simulink subsystem "ScanDc"  (R2025a)
settings: Solver=VariableStepAuto  StartTime=0.0  StopTime=10.0  RelTol=1e-3
model mask{F0=0, Theta0=0, Kp_LF=0, Ki_LF=0, Ts=0, Amplitudedc=scan.Vdc, Amplitude=0, Amplitude1=0, voltagedc=HVDC.Vdc, voltage=0, mva=0, f=scan.f, Tdis=scan.start, Tend=scan.end, T=1/scan.samplingfrequency}
  mask prompts: F0 "Initial frequency (Hz)"; Theta0 "Inital angle (deg)"; Kp_LF "Proportional gain"; Ki_LF "Integral gain"; Ts "Sample time (sec)"; Amplitudedc "DC voltage disturbance (PU)"; Amplitude "D axis voltage disturbance (PU)"; Amplitude1 "Q axis voltage disturbance (PU)"; voltagedc "Base DC Voltage (V)"; voltage "Base AC Voltage (V)"; mva "Base voltr ampere (VA)"; f "Disturbance Frequency (Hz)"; Tdis "Disturbance start time (sec)"; Tend "Disturbance end time (sec)"; T "Sample Time of PRBS (sec)"
undefined symbols (not defined in the file): DiscIntNeverNeededParam, ee_sli_rtmsupport, gcbh, w
libraries: slctrl_fre x6, eeGeneralControl x4, slctrl_signal x3, eeTransforms x2, ee_lib x1, nesl_utility x1, simulink x1
(part 1 of 2)
settings Model: Creator=rajarshd  LastModifiedBy=rajarshd

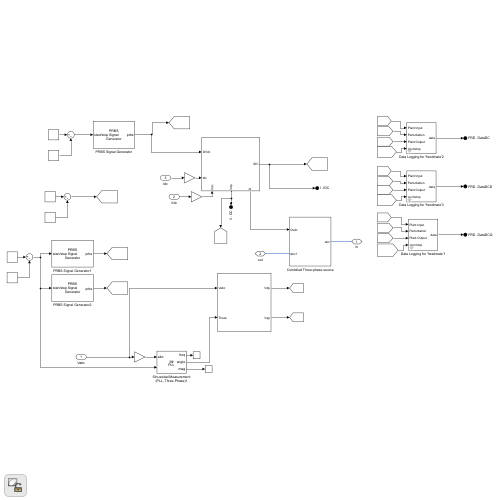
[thumbnail: Simulink's stored preview of the top-level diagram]
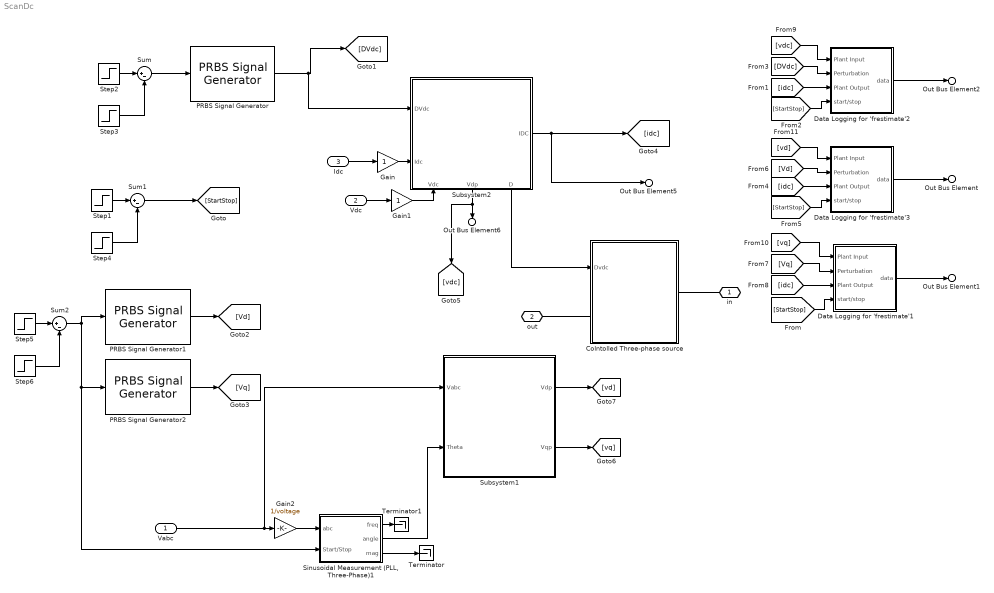
== system ScanDc ==
  Vabc : Inport
  Vdc : Inport  Port=2
  Idc : Inport  Port=3
  Colntolled Three-phase source : Subsystem
  Data Logging for 'frestimate'1 : Subsystem  mask(Companion Data Logger){Ts=T, SignalType=PRBS, Frequencies=[1:1:2e3], NumOfSetPeriod=1, NumOfEstPeriod=1, PRBSNumOfPeriod=1, ReadySignalActiveChoice=VariantPRBS, InfoSignalActiveChoice=VariantPRBS}
      mask prompts: Ts "Sample Time (Ts)"; SignalType "Input Signal Type"; Frequencies "Frequencies Vector"; NumOfSetPeriod "Number of Settling Periods"; NumOfEstPeriod "Number of Estimation Periods"; PRBSNumOfPeriod "Number of PRBS Signal Periods"; ReadySignalActiveChoice "Simulink:Variants:LabelComboBox"; InfoSignalActiveChoice "Simulink:Variants:LabelComboBox"
      mask help: Log data from signal generator blocks to work with "frestimate" API or frequency response estimation.
      mask init:
      | IsSinestreamSignal = strcmpi(get_param(gcb,'SignalType'),'Sinestream');
      |     IsPRBSSignal = strcmpi(get_param(gcb,'SignalType'),'PRBS');
      |     maskObj = Simulink.Mask.get(gcb);
      |     objectSinestream = maskObj.getDialogControl('SinestreamPanel');
      |     objectPRBS = maskObj.getDialogControl('PRBSPanel');
      |     %% Update optional inports
      |     inport_name = {'Frequency Index'};
      |     AvailableBlocks = get_param(gcb,'Blocks');
      |     % what exists in the block (old)
      |     type_in_block = ismember(inport_name,AvailableBlocks);
      |     % what is specified in the dialog (new)
      |     type_in_mask = IsSinestreamSignal;
      |     if IsSinestreamSignal
      |         objectSinestream.Visible = 'on';
      |         objectPRBS.Visible = 'off';
      |         set_param(gcb,'ReadySignalActiveChoice','VariantSinestream');  
      |         set_param(gcb,'InfoSignalActiveChoice','VariantSinestream');        
      |     elseif IsPRBSSignal
      |         objectSinestream.Visible = 'off';
      |         objectPRBS.Visible = 'on';
      |         set_param(gcb,'ReadySignalActiveChoice','VariantPRBS');  
      |         set_param(gcb,'InfoSignalActiveChoice','VariantPRBS');        
      |     end
      |     % Update Inport
      |     port = 5;
      |     port = slctrlblkdlgs.OnlinePIDTuner.utilUpdateInport(gcb,'RateTransition_idx',AvailableBlocks,type_in_mask,type_in_block,1,'Frequency Index',port,1,'Frequencies','double');
      mask TypeOptions SignalType: Sinestream | PRBS
      mask TypeOptions ReadySignalActiveChoice: Generate Ready Signal/LabelModeActiveChoice
      mask TypeOptions InfoSignalActiveChoice: Generate Info Signal/LabelModeActiveChoice
      mask DialogControl Container3 Prompt: Signal Specific Settings
      mask DialogControl ReadySignalActiveChoice Prompt: Label mode active choice:
      mask DialogControl InfoSignalActiveChoice Prompt: Label mode active choice:
  Data Logging for 'frestimate'2 : Subsystem  mask(Companion Data Logger){Ts=T, SignalType=PRBS, Frequencies=[1:1:2e3], NumOfSetPeriod=1, NumOfEstPeriod=1, PRBSNumOfPeriod=1, ReadySignalActiveChoice=VariantPRBS, InfoSignalActiveChoice=VariantPRBS}
      mask prompts: Ts "Sample Time (Ts)"; SignalType "Input Signal Type"; Frequencies "Frequencies Vector"; NumOfSetPeriod "Number of Settling Periods"; NumOfEstPeriod "Number of Estimation Periods"; PRBSNumOfPeriod "Number of PRBS Signal Periods"; ReadySignalActiveChoice "Simulink:Variants:LabelComboBox"; InfoSignalActiveChoice "Simulink:Variants:LabelComboBox"
      mask help: Log data from signal generator blocks to work with "frestimate" API or frequency response estimation.
      mask init: same as ScanDc/Data Logging for 'frestimate'1
      mask TypeOptions SignalType: Sinestream | PRBS
      mask TypeOptions ReadySignalActiveChoice: Generate Ready Signal/LabelModeActiveChoice
      mask TypeOptions InfoSignalActiveChoice: Generate Info Signal/LabelModeActiveChoice
      mask DialogControl Container3 Prompt: Signal Specific Settings
      mask DialogControl ReadySignalActiveChoice Prompt: Label mode active choice:
      mask DialogControl InfoSignalActiveChoice Prompt: Label mode active choice:
  Data Logging for 'frestimate'3 : Subsystem  mask(Companion Data Logger){Ts=T, SignalType=PRBS, Frequencies=[1:1:2e3], NumOfSetPeriod=1, NumOfEstPeriod=1, PRBSNumOfPeriod=1, ReadySignalActiveChoice=VariantPRBS, InfoSignalActiveChoice=VariantPRBS}
      mask prompts: Ts "Sample Time (Ts)"; SignalType "Input Signal Type"; Frequencies "Frequencies Vector"; NumOfSetPeriod "Number of Settling Periods"; NumOfEstPeriod "Number of Estimation Periods"; PRBSNumOfPeriod "Number of PRBS Signal Periods"; ReadySignalActiveChoice "Simulink:Variants:LabelComboBox"; InfoSignalActiveChoice "Simulink:Variants:LabelComboBox"
      mask help: Log data from signal generator blocks to work with "frestimate" API or frequency response estimation.
      mask init: same as ScanDc/Data Logging for 'frestimate'1
      mask TypeOptions SignalType: Sinestream | PRBS
      mask TypeOptions ReadySignalActiveChoice: Generate Ready Signal/LabelModeActiveChoice
      mask TypeOptions InfoSignalActiveChoice: Generate Info Signal/LabelModeActiveChoice
      mask DialogControl Container3 Prompt: Signal Specific Settings
      mask DialogControl ReadySignalActiveChoice Prompt: Label mode active choice:
      mask DialogControl InfoSignalActiveChoice Prompt: Label mode active choice:
  Gain : Gain
  Gain1 : Gain
  Gain2 : Gain  Gain=1/voltage
  PRBS Signal Generator : slctrl_signal/PRBS Signal Generator  DiscreteTs=T  BlockDataType=double  SignalSource=Block parameters  Frequencies=f*2*pi  FreqUnits=rad/s  Amplitudes=Amplitudedc*voltagedc+1e-9  NumOfFreq=3  NumOfPRBSPeriod=1  UseAutogenNumOfPRBSPeriod=off  PRBSSignalOrder=16  UseAutogenPRBSSignalOrder=on  UseExternalTs=off  CompiledTsChoice=InternalTs
      settings: LibrarySourceBlock=slctrlblks/Signal Generation/PRBS Signal Generator
  PRBS Signal Generator1 : slctrl_signal/PRBS Signal Generator  DiscreteTs=T  BlockDataType=double  SignalSource=Block parameters  Frequencies=f*2*pi  FreqUnits=rad/s  Amplitudes=Amplitude*voltage+1e-9  NumOfFreq=3  NumOfPRBSPeriod=1  UseAutogenNumOfPRBSPeriod=off  PRBSSignalOrder=16  UseAutogenPRBSSignalOrder=on  UseExternalTs=off  CompiledTsChoice=InternalTs
      settings: LibrarySourceBlock=slctrlblks/Signal Generation/PRBS Signal Generator
  PRBS Signal Generator2 : slctrl_signal/PRBS Signal Generator  DiscreteTs=T  BlockDataType=double  SignalSource=Block parameters  Frequencies=f*2*pi  FreqUnits=rad/s  Amplitudes=Amplitude1*voltage+1e-9  NumOfFreq=3  NumOfPRBSPeriod=1  UseAutogenNumOfPRBSPeriod=off  PRBSSignalOrder=16  UseAutogenPRBSSignalOrder=on  UseExternalTs=off  CompiledTsChoice=InternalTs
      settings: LibrarySourceBlock=slctrlblks/Signal Generation/PRBS Signal Generator
  "Sinusoidal Measurement (PLL, Three-Phase)1" : Subsystem  LoadFcn=ee_sli_rtmsupport( 'loadfcn', gcbh );  mask(Sinusoidal Measurement (PLL, Three-Phase)){Kp_LF=Kp_LF, Ki_LF=Ki_LF, F0=F0, Theta0=Theta0, Ts=Ts}
      mask prompts: Kp_LF "physmod:ee:library:comments:control:eeSinusoidalMeasurement:LoopFilterProportionalGain_MP"; Ki_LF "physmod:ee:library:comments:control:eeSinusoidalMeasurement:LoopFilterIntegralGain_MP"; F0 "physmod:ee:library:comments:control:eeSinusoidalMeasurement:InitialFrequencyHz_MP"; Theta0 "physmod:ee:library:comments:control:eeSinusoidalMeasurement:InitialPhaseAnglerad_MP"; Ts "physmod:ee:library:comments:control:eeSinusoidalMeasurement:SampleTime1ForInherited_MP"
      mask help: physmod:ee:library:comments:control:eeSinusoidalMeasurement:SinusoidalPowerMeasurementPLLThreePhase_MD
      mask init:
      | timeDomain = ee.mask.initializeThreePhaseSinusoidalMeasurementPLL(Ts);
      settings: CopyFcn=ee_sli_rtmsupport( 'copyfcn', gcbh );  DeleteFcn=ee_sli_rtmsupport( 'deletefcn', gcbh );  ModelCloseFcn=ee_sli_rtmsupport( 'modelclosefcn', gcbh );  PostSaveFcn=ee_sli_rtmsupport( 'postsavefcn', gcbh );  PreCopyFcn=ee_sli_rtmsupport( 'precopyfcn', gcbh );  OpenFcn=ee_sli_rtmsupport( 'openfcn', gcbh );  CloseFcn=ee_sli_rtmsupport( 'closefcn', gcbh );  PreDeleteFcn=ee_sli_rtmsupport( 'predeletefcn', gcbh );
      settings: LibrarySourceBlock=|
      | ee_sl_lib/Measurements/Sinusoidal Measurement
      | (PLL, Three-Phase)
      mask Help: web(nesl_help(gcbh))
      mask TypeOptions Ts:
      | Angle/Integrator with
      | Wrapped State
      | (Discrete or Continuous)/Ts | PI/Integrator
      | (Discrete or Continuous)/Ts | Moving Average
      | (Variable Frequency)/Ts | Low-Pass Filter
      | (Discrete or Continuous)/Ts
      mask DialogControl Kp_LF Prompt: Loop filter proportional gain
      mask DialogControl Ki_LF Prompt: Loop filter integral gain
      mask DialogControl F0 Prompt: Initial frequency (Hz)
      mask DialogControl Theta0 Prompt: Initial phase angle (rad)
      mask DialogControl Ts Prompt: Sample time (-1 for inherited)
      mask Display: ee.mask.drawThreePhaseSinusoidalMeasurementPLL;
  Step1 : Step  Time=Tdis-0.001  SampleTime=Ts
  Step2 : Step  Time=Tdis  SampleTime=Ts
  Step3 : Step  Time=Tend  SampleTime=Ts
  Step4 : Step  Time=Tend-0.001  SampleTime=Ts
  Step5 : Step  Time=Tdis  SampleTime=Ts
  Step6 : Step  Time=Tend  SampleTime=Ts
  Subsystem1 : Subsystem
      settings: PortSchema="{\"entries\":[{\"content\":{\"sides\":[{\"content\":{},\"type\":\"ConnectorPlacement.EquallySpacedRectSide\",\"uuid\":\"9594ab20-6a90-4061-9191-964719779161\"},{\"content\":{\"side\":\"RIGHT\"},\"type\":\"ConnectorPlacement.EquallySpacedRectSide\",\"uuid\":\"7728c146-30c2-48f5-81ca-653b56ee64fb\"},{\"content\":{\"connectorIds\":[\"Out1\",\"Out2\"],\"side\":\"TOP\"},\"type\":\"ConnectorPlacement.EquallySpacedRectSide\",\"uuid\":\"8060c2dd-01d9-4157-a0b3-59db77887fcf\"},{\"content\":{\"connectorIds\":[\"In1\",\"In2\"],\"side\":\"BOTTOM\"},\"type\":\"ConnectorPlacement.EquallySpacedRectSide\",\"uuid\":\"6c62adf9-210a-4ad7-b383-6cff41840c61\"}]},\"type\":\"ConnectorPlacement.EquallySpacedConnector\",\"uuid\":\"38a4dacf-dba1-4794-be83-b6cd11059d5d\"}],\"packageUris\":[\"http://schema.mathworks.com/mf0/Connector/R2020b\"],\"version\":\"1.0\"}"
  Subsystem2 : Subsystem
      settings: PortSchema="{\"entries\":[{\"content\":{\"sides\":[{\"content\":{\"connectorIds\":[\"In1\",\"In2\"]},\"type\":\"ConnectorPlacement.EquallySpacedRectSide\",\"uuid\":\"9594ab20-6a90-4061-9191-964719779161\"},{\"content\":{\"connectorIds\":[\"Out1\"],\"side\":\"RIGHT\"},\"type\":\"ConnectorPlacement.EquallySpacedRectSide\",\"uuid\":\"7728c146-30c2-48f5-81ca-653b56ee64fb\"},{\"content\":{\"side\":\"TOP\"},\"type\":\"ConnectorPlacement.EquallySpacedRectSide\",\"uuid\":\"8060c2dd-01d9-4157-a0b3-59db77887fcf\"},{\"content\":{\"connectorIds\":[\"In3\",\"Out2\",\"Out3\"],\"side\":\"BOTTOM\"},\"type\":\"ConnectorPlacement.EquallySpacedRectSide\",\"uuid\":\"6c62adf9-210a-4ad7-b383-6cff41840c61\"}]},\"type\":\"ConnectorPlacement.EquallySpacedConnector\",\"uuid\":\"38a4dacf-dba1-4794-be83-b6cd11059d5d\"}],\"packageUris\":[\"http://schema.mathworks.com/mf0/Connector/R2020b\"],\"version\":\"1.0\"}"
  Sum : Sum  Inputs=|+-
  Sum1 : Sum  Inputs=|+-
  Sum2 : Sum  Inputs=|+-
  Terminator : Terminator
  Terminator1 : Terminator
  in : PMIOPort  Side=Left
  out : PMIOPort  Port=2  Side=Right
  Out Bus Element5 : Outport  PortName=I  Element=IDC
  Out Bus Element6 : Outport  Port=2  PortName=V  Element=DC
  Out Bus Element : Outport  Port=3  PortName=FRD  Element=DataDCD
  Out Bus Element1 : Outport  Port=3  PortName=FRD  Element=DataDCQ
  Out Bus Element2 : Outport  Port=3  PortName=FRD  Element=DataDC
  wires:
  PRBS Signal Generator/1 -> [DVdc], Subsystem2/1(DVdc)
  Sum2/1 -> PRBS Signal Generator1/1, "Sinusoidal Measurement (PLL, Three-Phase)1"/2(Start/Stop), PRBS Signal Generator2/1
  Subsystem2/2(Vdp) -> Out Bus Element6/1, [vdc]
  Sum/1 -> PRBS Signal Generator/1
  Step2/1 -> Sum/1
  Step3/1 -> Sum/2
  Sum1/1 -> [StartStop]
  Step1/1 -> Sum1/1
  Step4/1 -> Sum1/2
  Step6/1 -> Sum2/2
  Step5/1 -> Sum2/1
  PRBS Signal Generator1/1 -> [Vd]
  PRBS Signal Generator2/1 -> [Vq]
  Vdc/1 -> Gain1/1
  Subsystem2/3(D) -> Colntolled Three-phase source/1(Dvdc)
  "Sinusoidal Measurement (PLL, Three-Phase)1"/2(angle) -> Subsystem1/2(Theta)
  "Sinusoidal Measurement (PLL, Three-Phase)1"/1(freq) -> Terminator1/1
  "Sinusoidal Measurement (PLL, Three-Phase)1"/3(mag) -> Terminator/1
  [vd] -> Data Logging for 'frestimate'3/1(Plant Input)
  [Vd] -> Data Logging for 'frestimate'3/2(Perturbation)
  [idc] -> Data Logging for 'frestimate'3/3(Plant Output)
  [StartStop] -> Data Logging for 'frestimate'3/4(start/stop)
  Data Logging for 'frestimate'1/1(data) -> Out Bus Element1/1
  Data Logging for 'frestimate'3/1(data) -> Out Bus Element/1
  Data Logging for 'frestimate'2/1(data) -> Out Bus Element2/1
  [vq] -> Data Logging for 'frestimate'1/1(Plant Input)
  [Vq] -> Data Logging for 'frestimate'1/2(Perturbation)
  [idc] -> Data Logging for 'frestimate'1/3(Plant Output)
  [StartStop] -> Data Logging for 'frestimate'1/4(start/stop)
  [vdc] -> Data Logging for 'frestimate'2/1(Plant Input)
  [DVdc] -> Data Logging for 'frestimate'2/2(Perturbation)
  [idc] -> Data Logging for 'frestimate'2/3(Plant Output)
  [StartStop] -> Data Logging for 'frestimate'2/4(start/stop)
  Subsystem1/1(Vdp) -> [vd]
  Subsystem1/2(Vqp) -> [vq]
  Subsystem2/1(IDC) -> Out Bus Element5/1, [idc]
  Vabc/1 -> Subsystem1/1(Vabc), Gain2/1
  Gain/1 -> Subsystem2/2(Idc)
  Idc/1 -> Gain/1
  Gain1/1 -> Subsystem2/3(Vdc)
  Gain2/1 -> "Sinusoidal Measurement (PLL, Three-Phase)1"/1(abc)
  connections:
  Colntolled Three-phase source/RConn1 -- in/RConn1
  out/RConn1 -- Colntolled Three-phase source/LConn1

== system ScanDc/Colntolled Three-phase source ==
  Dvdc : Inport
  Programmable Voltage Source2 : ee_lib/Sources/Programmable Voltage Source  magnitude_type=ee.enum.timechanging.constant  ac_magnitude=0 V  magn_ramp=1 V/s  magn_step=1 V  magn_modu_magn=1 V  magn_modu_freq=1 Hz  magn_t1=1 s  magn_t2=2 s  frequency_type=ee.enum.timechanging.constant  ac_frequency=60 Hz  freq_ramp=1 Hz/s  freq_step=1 Hz  freq_modu_magn=1 Hz  freq_modu_freq=1 Hz  freq_t1=1 s  freq_t2=2 s  phase_type=ee.enum.timechanging.constant  ac_shift=0 deg  phase_ramp=1 deg/s  phase_step=1 deg  phase_modu_magn=1 deg  phase_modu_freq=1 Hz  phase_t1=1 s  phase_t2=2 s  dc_type=ee.enum.timechanging.external  dc_voltage=0 V  dc_ramp=1 V/s  dc_step=1 V  dc_modu_magn=1 V  dc_modu_freq=1 Hz  dc_t1=1 s  dc_t2=2 s  harmonic_option=0  harmonic_orders=[5, 7, 11, 13]  harmonic_ratios=[.1, .1, .1, .1]  harmonic_shifts=[0, 0, 0, 0] deg  harmonic_t1=-inf s  harmonic_t2=inf s  noise_mode=0  PSD=0 V^2/Hz  repeatability=1  auto_seed=0  user_seed=0  sample_time=1e-3 s  i_specify=off  i_priority=None  i=0 A  i_nominal_specify=off  i_nominal_value=1  i_nominal_unit=A  v_specify=off  v_priority=None  v=0 V  v_nominal_specify=off  v_nominal_value=1  v_nominal_unit=V
      settings: InternalSimscapePortConfiguration="{\"Bottom\":[],\"Left\":[{\"id\":\"p\",\"label\":\"+\",\"type\":\"foundation.electrical.electrical\"}],\"Right\":[{\"id\":\"ext_dc\",\"label\":\"DC\",\"type\":\"input\"},{\"id\":\"n\",\"label\":\"-\",\"type\":\"foundation.electrical.electrical\"}],\"Top\":[]}"
  Simulink-PS Converter : nesl_utility/Simulink-PS Converter  PhysicalDomain=network_engine_domain  SubClassName=ps_input  LeftPortType=input  RightPortType=output  PseudoPeriodic=off  Frequencies=[]  NoiseDistribution=none  NoiseParameters=[]  Unit=1  AffineConversion=off  FilteringAndDerivatives=provide  SimscapeFilterOrder=1  InputFilterTimeConstant=0.001  UdotUserProvided=0
  abc1 : PMIOPort  Side=Left
  abc : PMIOPort  Port=2  Side=Right
  wires:
  Dvdc/1 -> Simulink-PS Converter/1
  connections:
  Programmable Voltage Source2/LConn1 -- abc1/RConn1
  Simulink-PS Converter/RConn1 -- Programmable Voltage Source2/RConn1
  Programmable Voltage Source2/RConn2 -- abc/RConn1

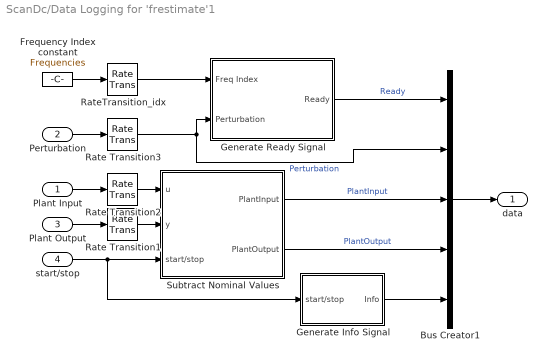
== system ScanDc/Data Logging for 'frestimate'1 ==
  Plant Input : Inport
  Perturbation : Inport  Port=2
  Plant Output : Inport  Port=3
  start/stop : Inport  Port=4
  Bus Creator1 : BusCreator  Inputs=5
  Frequency Index constant : Constant  Value=Frequencies  OutDataTypeStr=double
  Generate Info Signal : Subsystem  Variant=on  VariantControlMode=label  LabelModeActiveChoice=VariantPRBS
  Generate Ready Signal : Subsystem  Variant=on  VariantControlMode=label  LabelModeActiveChoice=VariantPRBS
  Rate Transition1 : RateTransition  OutPortSampleTime=Ts
  Rate Transition2 : RateTransition  OutPortSampleTime=Ts
  Rate Transition3 : RateTransition  OutPortSampleTime=Ts
  RateTransition_idx : RateTransition  OutPortSampleTime=Ts
  Subtract Nominal Values : Subsystem
  data : Outport
  wires:
  Frequency Index constant/1 -> RateTransition_idx/1
  RateTransition_idx/1 -> Generate Ready Signal/1(Freq Index)
  Perturbation/1 -> Rate Transition3/1
  Rate Transition1/1 -> Subtract Nominal Values/2(y)
  Rate Transition2/1 -> Subtract Nominal Values/1(u)
  start/stop/1 -> Subtract Nominal Values/3(start/stop), Generate Info Signal/1(start/stop)
  Plant Input/1 -> Rate Transition2/1
  Plant Output/1 -> Rate Transition1/1
  Generate Ready Signal/1(Ready) -> Bus Creator1/1  "Ready"
  Subtract Nominal Values/2(PlantOutput) -> Bus Creator1/4  "PlantOutput"
  Subtract Nominal Values/1(PlantInput) -> Bus Creator1/3  "PlantInput"
  Rate Transition3/1 -> Bus Creator1/2, Generate Ready Signal/2(Perturbation)  "Perturbation"
  Bus Creator1/1 -> data/1
  Generate Info Signal/1(Info) -> Bus Creator1/5

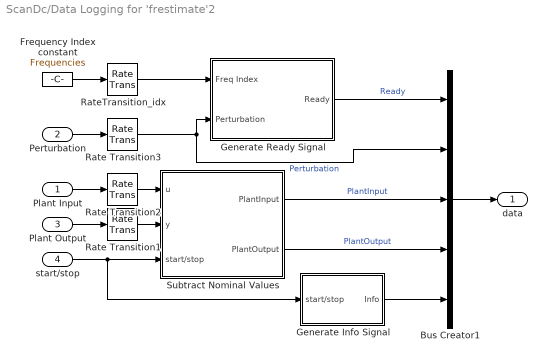
== system ScanDc/Data Logging for 'frestimate'2 ==
  Plant Input : Inport
  Perturbation : Inport  Port=2
  Plant Output : Inport  Port=3
  start/stop : Inport  Port=4
  Bus Creator1 : BusCreator  Inputs=5
  Frequency Index constant : Constant  Value=Frequencies  OutDataTypeStr=double
  Generate Info Signal : Subsystem  Variant=on  VariantControlMode=label  LabelModeActiveChoice=VariantPRBS
  Generate Ready Signal : Subsystem  Variant=on  VariantControlMode=label  LabelModeActiveChoice=VariantPRBS
  Rate Transition1 : RateTransition  OutPortSampleTime=Ts
  Rate Transition2 : RateTransition  OutPortSampleTime=Ts
  Rate Transition3 : RateTransition  OutPortSampleTime=Ts
  RateTransition_idx : RateTransition  OutPortSampleTime=Ts
  Subtract Nominal Values : Subsystem
  data : Outport
  wires:
  Frequency Index constant/1 -> RateTransition_idx/1
  RateTransition_idx/1 -> Generate Ready Signal/1(Freq Index)
  Perturbation/1 -> Rate Transition3/1
  Rate Transition1/1 -> Subtract Nominal Values/2(y)
  Rate Transition2/1 -> Subtract Nominal Values/1(u)
  start/stop/1 -> Subtract Nominal Values/3(start/stop), Generate Info Signal/1(start/stop)
  Plant Input/1 -> Rate Transition2/1
  Plant Output/1 -> Rate Transition1/1
  Generate Ready Signal/1(Ready) -> Bus Creator1/1  "Ready"
  Subtract Nominal Values/2(PlantOutput) -> Bus Creator1/4  "PlantOutput"
  Subtract Nominal Values/1(PlantInput) -> Bus Creator1/3  "PlantInput"
  Rate Transition3/1 -> Bus Creator1/2, Generate Ready Signal/2(Perturbation)  "Perturbation"
  Bus Creator1/1 -> data/1
  Generate Info Signal/1(Info) -> Bus Creator1/5

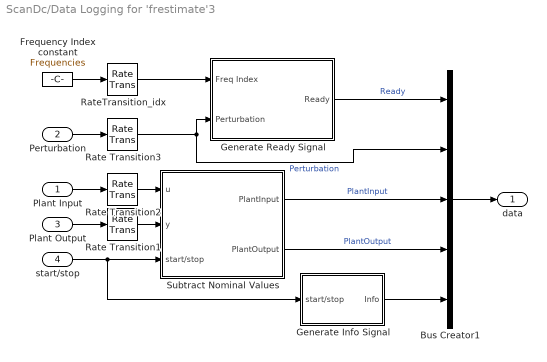
== system ScanDc/Data Logging for 'frestimate'3 ==
  Plant Input : Inport
  Perturbation : Inport  Port=2
  Plant Output : Inport  Port=3
  start/stop : Inport  Port=4
  Bus Creator1 : BusCreator  Inputs=5
  Frequency Index constant : Constant  Value=Frequencies  OutDataTypeStr=double
  Generate Info Signal : Subsystem  Variant=on  VariantControlMode=label  LabelModeActiveChoice=VariantPRBS
  Generate Ready Signal : Subsystem  Variant=on  VariantControlMode=label  LabelModeActiveChoice=VariantPRBS
  Rate Transition1 : RateTransition  OutPortSampleTime=Ts
  Rate Transition2 : RateTransition  OutPortSampleTime=Ts
  Rate Transition3 : RateTransition  OutPortSampleTime=Ts
  RateTransition_idx : RateTransition  OutPortSampleTime=Ts
  Subtract Nominal Values : Subsystem
  data : Outport
  wires:
  Frequency Index constant/1 -> RateTransition_idx/1
  RateTransition_idx/1 -> Generate Ready Signal/1(Freq Index)
  Perturbation/1 -> Rate Transition3/1
  Rate Transition1/1 -> Subtract Nominal Values/2(y)
  Rate Transition2/1 -> Subtract Nominal Values/1(u)
  start/stop/1 -> Subtract Nominal Values/3(start/stop), Generate Info Signal/1(start/stop)
  Plant Input/1 -> Rate Transition2/1
  Plant Output/1 -> Rate Transition1/1
  Generate Ready Signal/1(Ready) -> Bus Creator1/1  "Ready"
  Subtract Nominal Values/2(PlantOutput) -> Bus Creator1/4  "PlantOutput"
  Subtract Nominal Values/1(PlantInput) -> Bus Creator1/3  "PlantInput"
  Rate Transition3/1 -> Bus Creator1/2, Generate Ready Signal/2(Perturbation)  "Perturbation"
  Bus Creator1/1 -> data/1
  Generate Info Signal/1(Info) -> Bus Creator1/5

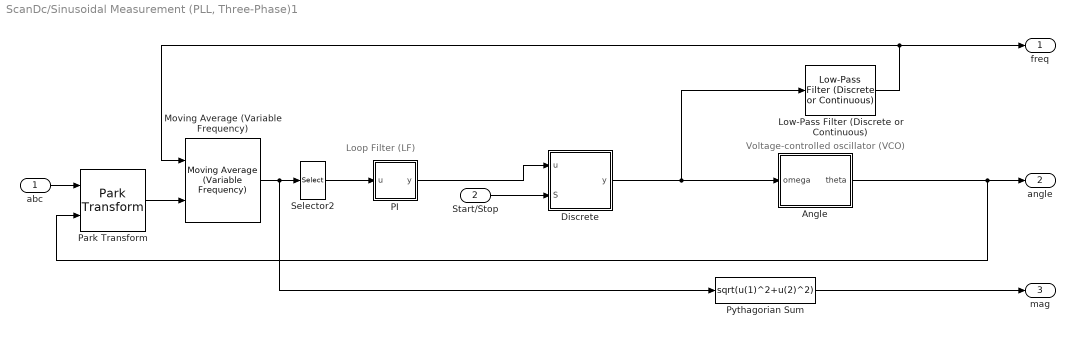
== system ScanDc/Sinusoidal Measurement (PLL, Three-Phase)1 ==
  note: Loop Filter (LF)
  note: Voltage-controlled oscillator (VCO)
  abc : Inport  PortDimensions=3  SampleTime=Ts
  Start/Stop : Inport  Port=2
  Angle : Subsystem
  Discrete : Subsystem  VariantControl=Discrete
      settings: LibrarySourceBlock=eeGeneralControl/Signal Sample and Hold/Discrete
  Low-Pass Filter (Discrete or Continuous) : eeGeneralControl/Low-Pass Filter (Discrete or Continuous)  K=1/2/pi  T=1e-3  B=inf  A=-inf  init_option=Specify as parameter  x0=F0  Ts=Ts
  Moving Average (Variable Frequency) : eeGeneralControl/Moving Average (Variable Frequency)  VariantControl=Variant1  LabelModeActiveChoice=Discrete  f0=F0  fmin=5  x0=0  BufferSize=8192  Ts=Ts
  PI : Subsystem
  Park Transform : eeTransforms/Park Transform  AxisAlignment=Q-axis  PowerInvariant=on
  Pythagorian Sum : Fcn  Expr=sqrt(u(1)^2+u(2)^2)
  Selector2 : Selector  InputPortWidth=3  IndexOptions=Index vector (dialog)  Indices=[2]  OutputSizes=1
  freq : Outport  VectorParamsAs1DForOutWhenUnconnected=off
  angle : Outport  Port=2  VectorParamsAs1DForOutWhenUnconnected=off
  mag : Outport  Port=3  VectorParamsAs1DForOutWhenUnconnected=off
  wires:
  Discrete/1(y) -> Angle/1(omega), Low-Pass Filter (Discrete or Continuous)/1
  PI/1(y) -> Discrete/1(u)
  Start/Stop/1 -> Discrete/2(S)
  Moving Average (Variable Frequency)/1 -> Selector2/1, Pythagorian Sum/1
  Selector2/1 -> PI/1(u)
  Low-Pass Filter (Discrete or Continuous)/1 -> freq/1, Moving Average (Variable Frequency)/1
  Angle/1(theta) -> angle/1, Park Transform/2
  Park Transform/1 -> Moving Average (Variable Frequency)/2
  Pythagorian Sum/1 -> mag/1
  abc/1 -> Park Transform/1

== system ScanDc/Subsystem1 ==
  Vabc : Inport
  Theta : Inport  Port=2
  Demux1 : Demux  Outputs=3
  Park Transform1 : eeTransforms/Park Transform  AxisAlignment=Q-axis  PowerInvariant=on
  Terminator1 : Terminator
  Vdp : Outport
  Vqp : Outport  Port=2
  wires:
  Park Transform1/1 -> Demux1/1
  Demux1/2 -> Vqp/1
  Demux1/1 -> Vdp/1
  Demux1/3 -> Terminator1/1
  Vabc/1 -> Park Transform1/1
  Theta/1 -> Park Transform1/2

== system ScanDc/Subsystem2 ==
  DVdc : Inport
  Idc : Inport  Port=2
  Vdc : Inport  Port=3
  IDC : Outport
  Vdp : Outport  Port=2
  D : Outport  Port=3
  wires:
  Vdc/1 -> Vdp/1
  DVdc/1 -> D/1
  Idc/1 -> IDC/1

== system ScanDc/Data Logging for 'frestimate'1/Generate Info Signal ==
  note: 1) Add Subsystem or Model blocks as valid variant choices.
      | 2) You cannot connect blocks at this level. At simulation, connectivity is automatically
      | determined, based on the active variant and port name matching.
  start/stop : Inport
  PRBS : Subsystem  VariantControl=VariantPRBS
  Sinestream : Subsystem  VariantControl=VariantSinestream
  Info : Outport

== system ScanDc/Data Logging for 'frestimate'1/Generate Ready Signal ==
  note: 1) Add Subsystem or Model blocks as valid variant choices.
      | 2) You cannot connect blocks at this level. At simulation, connectivity is automatically
      | determined, based on the active variant and port name matching.
  Freq Index : Inport
  Perturbation : Inport  Port=2
  PRBS : Subsystem  VariantControl=VariantPRBS
  Sinestream : Subsystem  VariantControl=VariantSinestream
  Ready : Outport

== system ScanDc/Data Logging for 'frestimate'1/Subtract Nominal Values ==
  u : Inport
  y : Inport  Port=2
  start/stop : Inport  Port=3
  Enabled Subsystem : Subsystem  TreatAsAtomicUnit=on
  PlantInput : Outport
  PlantOutput : Outport  Port=2
  wires:
  Enabled Subsystem/2(PlantOutput) -> PlantOutput/1
  Enabled Subsystem/1(PlantInput) -> PlantInput/1
  start/stop/1 -> Enabled Subsystem/Enable, Enabled Subsystem/3(start/stop)
  y/1 -> Enabled Subsystem/2(y)
  u/1 -> Enabled Subsystem/1(u)

== system ScanDc/Data Logging for 'frestimate'2/Generate Info Signal ==
  note: 1) Add Subsystem or Model blocks as valid variant choices.
      | 2) You cannot connect blocks at this level. At simulation, connectivity is automatically
      | determined, based on the active variant and port name matching.
  start/stop : Inport
  PRBS : Subsystem  VariantControl=VariantPRBS
  Sinestream : Subsystem  VariantControl=VariantSinestream
  Info : Outport

== system ScanDc/Data Logging for 'frestimate'2/Generate Ready Signal ==
  note: 1) Add Subsystem or Model blocks as valid variant choices.
      | 2) You cannot connect blocks at this level. At simulation, connectivity is automatically
      | determined, based on the active variant and port name matching.
  Freq Index : Inport
  Perturbation : Inport  Port=2
  PRBS : Subsystem  VariantControl=VariantPRBS
  Sinestream : Subsystem  VariantControl=VariantSinestream
  Ready : Outport

== system ScanDc/Data Logging for 'frestimate'2/Subtract Nominal Values ==
  u : Inport
  y : Inport  Port=2
  start/stop : Inport  Port=3
  Enabled Subsystem : Subsystem  TreatAsAtomicUnit=on
  PlantInput : Outport
  PlantOutput : Outport  Port=2
  wires:
  Enabled Subsystem/2(PlantOutput) -> PlantOutput/1
  Enabled Subsystem/1(PlantInput) -> PlantInput/1
  start/stop/1 -> Enabled Subsystem/Enable, Enabled Subsystem/3(start/stop)
  y/1 -> Enabled Subsystem/2(y)
  u/1 -> Enabled Subsystem/1(u)

== system ScanDc/Data Logging for 'frestimate'3/Generate Info Signal ==
  note: 1) Add Subsystem or Model blocks as valid variant choices.
      | 2) You cannot connect blocks at this level. At simulation, connectivity is automatically
      | determined, based on the active variant and port name matching.
  start/stop : Inport
  PRBS : Subsystem  VariantControl=VariantPRBS
  Sinestream : Subsystem  VariantControl=VariantSinestream
  Info : Outport

== system ScanDc/Data Logging for 'frestimate'3/Generate Ready Signal ==
  note: 1) Add Subsystem or Model blocks as valid variant choices.
      | 2) You cannot connect blocks at this level. At simulation, connectivity is automatically
      | determined, based on the active variant and port name matching.
  Freq Index : Inport
  Perturbation : Inport  Port=2
  PRBS : Subsystem  VariantControl=VariantPRBS
  Sinestream : Subsystem  VariantControl=VariantSinestream
  Ready : Outport

== system ScanDc/Data Logging for 'frestimate'3/Subtract Nominal Values ==
  u : Inport
  y : Inport  Port=2
  start/stop : Inport  Port=3
  Enabled Subsystem : Subsystem  TreatAsAtomicUnit=on
  PlantInput : Outport
  PlantOutput : Outport  Port=2
  wires:
  Enabled Subsystem/2(PlantOutput) -> PlantOutput/1
  Enabled Subsystem/1(PlantInput) -> PlantInput/1
  start/stop/1 -> Enabled Subsystem/Enable, Enabled Subsystem/3(start/stop)
  y/1 -> Enabled Subsystem/2(y)
  u/1 -> Enabled Subsystem/1(u)

== system ScanDc/Sinusoidal Measurement (PLL, Three-Phase)1/Angle ==
  omega : Inport
  Integrator with Wrapped State (Discrete or Continuous) : eeGeneralControl/Integrator with Wrapped State (Discrete or Continuous)  LabelModeActiveChoice=Continuous  WrappedStateUpperValue=2*pi  WrappedStateLowerValue=0  x0=Theta0  Ts=Ts
  theta : Outport  VectorParamsAs1DForOutWhenUnconnected=off
  wires:
  Integrator with Wrapped State (Discrete or Continuous)/1 -> theta/1
  omega/1 -> Integrator with Wrapped State (Discrete or Continuous)/1

== system ScanDc/Sinusoidal Measurement (PLL, Three-Phase)1/Discrete ==
  u : Inport  SampleTime=Ts
  S : Inport  Port=2  SampleTime=Ts
  Data Type Conversion : DataTypeConversion  OutDataTypeStr=boolean  SaturateOnIntegerOverflow=off  RndMeth=Floor
  Delay : Delay  DelayLength=1  InitialCondition=0
  Switch : Switch  Criteria=u2 ~= 0  SaturateOnIntegerOverflow=off  InputSameDT=off
  y : Outport  VectorParamsAs1DForOutWhenUnconnected=off
  wires:
  u/1 -> Switch/3
  Delay/1 -> Switch/1
  Switch/1 -> y/1, Delay/1
  Data Type Conversion/1 -> Switch/2
  S/1 -> Data Type Conversion/1

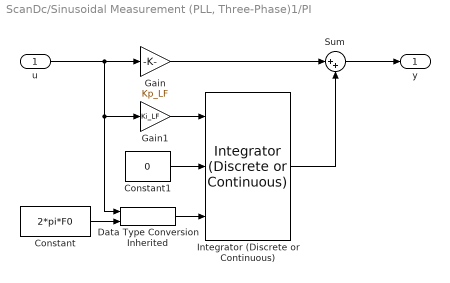
== system ScanDc/Sinusoidal Measurement (PLL, Three-Phase)1/PI ==
  u : Inport
  Constant : Constant  Value=2*pi*F0  SampleTime=Ts
  Constant1 : Constant  Value=0  SampleTime=Ts
  Data Type Conversion Inherited : simulink/Signal Attributes/Data Type Conversion Inherited  ConvertRealWorld=Real World Value  DoSatur=off
  Gain : Gain  Gain=Kp_LF
  Gain1 : Gain  Gain=Ki_LF
  Integrator (Discrete or Continuous) : eeGeneralControl/Integrator (Discrete or Continuous)  LabelModeActiveChoice=Continuous  IntegratorMethod=Integration: Forward Euler  ExternalReset=level  LimitType=Anti-windup  B=inf  A=-inf  Ts=Ts
  Sum : Sum  Inputs=|++
  y : Outport  VectorParamsAs1DForOutWhenUnconnected=off
  wires:
  Constant/1 -> Data Type Conversion Inherited/2
  Data Type Conversion Inherited/1 -> Integrator (Discrete or Continuous)/3
  Gain1/1 -> Integrator (Discrete or Continuous)/1
  u/1 -> Gain1/1, Data Type Conversion Inherited/1, Gain/1
  Gain/1 -> Sum/1
  Integrator (Discrete or Continuous)/1 -> Sum/2
  Sum/1 -> y/1
  Constant1/1 -> Integrator (Discrete or Continuous)/2

== system ScanDc/Data Logging for 'frestimate'1/Generate Info Signal/PRBS ==
  start/stop : Inport
  Info Bus : BusCreator  Inputs=1
  Info Snapshot : slctrl_fre/Frequency Response Estimator/Frequency Response Estimator/Variant Subsystem/PRBSNoEst/Info Snapshot  SystemSampleTime=-1  VariantActivationTime=update diagram  EmptyChoice=off  PassThrough=off  PassThroughVariantControl=(default)  EmptyChoiceVariantControl=(default)  AllowFlexibleInterface=on  Latency=0  AutoFrameSizeCalculation=off
  PRBSNumPeriods : Constant  SampleTime=Ts
  Info : Outport
  wires:
  PRBSNumPeriods/1 -> Info Snapshot/1
  Info Bus/1 -> Info/1  "Info"
  Info Snapshot/1 -> Info Bus/1  "PRBSNumPeriods"
  start/stop/1 -> Info Snapshot/Enable

== system ScanDc/Data Logging for 'frestimate'1/Generate Info Signal/Sinestream ==
  start/stop : Inport
  Info Bus : BusCreator  Inputs=1
  Info Snapshot : slctrl_fre/Frequency Response Estimator/Frequency Response Estimator/Variant Subsystem/PRBSNoEst/Info Snapshot  SystemSampleTime=-1  VariantActivationTime=update diagram  EmptyChoice=off  PassThrough=off  PassThroughVariantControl=(default)  EmptyChoiceVariantControl=(default)  AllowFlexibleInterface=on  Latency=0  AutoFrameSizeCalculation=off
  frequencies : Constant  Value=w  SampleTime=Ts
  Info : Outport
  wires:
  Info Snapshot/1 -> Info Bus/1  "frequencies"
  frequencies/1 -> Info Snapshot/1
  start/stop/1 -> Info Snapshot/Enable
  Info Bus/1 -> Info/1  "Info"

== system ScanDc/Data Logging for 'frestimate'1/Generate Ready Signal/PRBS ==
  Freq Index : Inport
  Perturbation : Inport  Port=2
  Constant : Constant  Value=0  SampleTime=Ts
  Relational Operator : RelationalOperator  Operator=~=  OutDataTypeStr=boolean  RndMeth=Simplest  InputSameDT=off
  Terminator : Terminator
  Ready : Outport
  wires:
  Relational Operator/1 -> Ready/1  "Ready"
  Constant/1 -> Relational Operator/2
  Perturbation/1 -> Relational Operator/1  "Perturbation"
  Freq Index/1 -> Terminator/1

== system ScanDc/Data Logging for 'frestimate'1/Generate Ready Signal/Sinestream ==
  Freq Index : Inport
  Perturbation : Inport  Port=2
  ExtractReadySignal : Subsystem  mask(Extract Ready Signal){Ts=Ts, Frequencies=w, NumOfSetPeriod=1, NumOfEstPeriod=2}
      mask prompts: Ts "Sample Time (Ts)"; Frequencies "Frequencies Vector"; NumOfSetPeriod "Number of Settling Periods"; NumOfEstPeriod "Number of Estimation Periods"
      mask help: Extract ready signal for the Sinestream Signal Generator block for offline frequency response estimation.
      mask init:
      | nw = length(Frequencies);
  Terminator : Terminator
  Ready : Outport
  wires:
  Freq Index/1 -> ExtractReadySignal/1(Frequency Index)
  Perturbation/1 -> Terminator/1
  ExtractReadySignal/1(Ready Signal) -> Ready/1  "Ready"

== system ScanDc/Data Logging for 'frestimate'1/Subtract Nominal Values/Enabled Subsystem ==
  u : Inport
  y : Inport  Port=2
  start/stop : Inport  Port=3
  Enable : EnablePort
  ExtractNominalValues : Subsystem  mask(Remove Nominal Signal){Ts=Ts}
      mask prompts: Ts "Samplt Time (sec)"
      mask help: Remove nominal baseline signal from logged data.
  Sum : Sum  Inputs=|+-
  Sum1 : Sum  Inputs=-+|
  PlantInput : Outport
  PlantOutput : Outport  Port=2
  wires:
  Sum1/1 -> PlantOutput/1
  y/1 -> ExtractNominalValues/2(y), Sum1/2
  ExtractNominalValues/2(yNominal) -> Sum1/1
  u/1 -> ExtractNominalValues/1(u), Sum/1
  ExtractNominalValues/1(uNominal) -> Sum/2
  Sum/1 -> PlantInput/1
  start/stop/1 -> ExtractNominalValues/3(start/stop)

== system ScanDc/Data Logging for 'frestimate'2/Generate Info Signal/PRBS ==
  start/stop : Inport
  Info Bus : BusCreator  Inputs=1
  Info Snapshot : slctrl_fre/Frequency Response Estimator/Frequency Response Estimator/Variant Subsystem/PRBSNoEst/Info Snapshot  SystemSampleTime=-1  VariantActivationTime=update diagram  EmptyChoice=off  PassThrough=off  PassThroughVariantControl=(default)  EmptyChoiceVariantControl=(default)  AllowFlexibleInterface=on  Latency=0  AutoFrameSizeCalculation=off
  PRBSNumPeriods : Constant  SampleTime=Ts
  Info : Outport
  wires:
  PRBSNumPeriods/1 -> Info Snapshot/1
  Info Bus/1 -> Info/1  "Info"
  Info Snapshot/1 -> Info Bus/1  "PRBSNumPeriods"
  start/stop/1 -> Info Snapshot/Enable

== system ScanDc/Data Logging for 'frestimate'2/Generate Info Signal/Sinestream ==
  start/stop : Inport
  Info Bus : BusCreator  Inputs=1
  Info Snapshot : slctrl_fre/Frequency Response Estimator/Frequency Response Estimator/Variant Subsystem/PRBSNoEst/Info Snapshot  SystemSampleTime=-1  VariantActivationTime=update diagram  EmptyChoice=off  PassThrough=off  PassThroughVariantControl=(default)  EmptyChoiceVariantControl=(default)  AllowFlexibleInterface=on  Latency=0  AutoFrameSizeCalculation=off
  frequencies : Constant  Value=w  SampleTime=Ts
  Info : Outport
  wires:
  Info Snapshot/1 -> Info Bus/1  "frequencies"
  frequencies/1 -> Info Snapshot/1
  start/stop/1 -> Info Snapshot/Enable
  Info Bus/1 -> Info/1  "Info"

== system ScanDc/Data Logging for 'frestimate'2/Generate Ready Signal/PRBS ==
  Freq Index : Inport
  Perturbation : Inport  Port=2
  Constant : Constant  Value=0  SampleTime=Ts
  Relational Operator : RelationalOperator  Operator=~=  OutDataTypeStr=boolean  RndMeth=Simplest  InputSameDT=off
  Terminator : Terminator
  Ready : Outport
  wires:
  Relational Operator/1 -> Ready/1  "Ready"
  Constant/1 -> Relational Operator/2
  Perturbation/1 -> Relational Operator/1  "Perturbation"
  Freq Index/1 -> Terminator/1

== system ScanDc/Data Logging for 'frestimate'2/Generate Ready Signal/Sinestream ==
  Freq Index : Inport
  Perturbation : Inport  Port=2
  ExtractReadySignal : Subsystem  mask(Extract Ready Signal){Ts=Ts, Frequencies=w, NumOfSetPeriod=1, NumOfEstPeriod=2}
      mask prompts: Ts "Sample Time (Ts)"; Frequencies "Frequencies Vector"; NumOfSetPeriod "Number of Settling Periods"; NumOfEstPeriod "Number of Estimation Periods"
      mask help: Extract ready signal for the Sinestream Signal Generator block for offline frequency response estimation.
      mask init:
      | nw = length(Frequencies);
  Terminator : Terminator
  Ready : Outport
  wires:
  Freq Index/1 -> ExtractReadySignal/1(Frequency Index)
  Perturbation/1 -> Terminator/1
  ExtractReadySignal/1(Ready Signal) -> Ready/1  "Ready"

== system ScanDc/Data Logging for 'frestimate'2/Subtract Nominal Values/Enabled Subsystem ==
  u : Inport
  y : Inport  Port=2
  start/stop : Inport  Port=3
  Enable : EnablePort
  ExtractNominalValues : Subsystem  mask(Remove Nominal Signal){Ts=Ts}
      mask prompts: Ts "Samplt Time (sec)"
      mask help: Remove nominal baseline signal from logged data.
  Sum : Sum  Inputs=|+-
  Sum1 : Sum  Inputs=-+|
  PlantInput : Outport
  PlantOutput : Outport  Port=2
  wires:
  Sum1/1 -> PlantOutput/1
  y/1 -> ExtractNominalValues/2(y), Sum1/2
  ExtractNominalValues/2(yNominal) -> Sum1/1
  u/1 -> ExtractNominalValues/1(u), Sum/1
  ExtractNominalValues/1(uNominal) -> Sum/2
  Sum/1 -> PlantInput/1
  start/stop/1 -> ExtractNominalValues/3(start/stop)

== system ScanDc/Data Logging for 'frestimate'3/Generate Info Signal/PRBS ==
  start/stop : Inport
  Info Bus : BusCreator  Inputs=1
  Info Snapshot : slctrl_fre/Frequency Response Estimator/Frequency Response Estimator/Variant Subsystem/PRBSNoEst/Info Snapshot  SystemSampleTime=-1  VariantActivationTime=update diagram  EmptyChoice=off  PassThrough=off  PassThroughVariantControl=(default)  EmptyChoiceVariantControl=(default)  AllowFlexibleInterface=on  Latency=0  AutoFrameSizeCalculation=off
  PRBSNumPeriods : Constant  SampleTime=Ts
  Info : Outport
  wires:
  PRBSNumPeriods/1 -> Info Snapshot/1
  Info Bus/1 -> Info/1  "Info"
  Info Snapshot/1 -> Info Bus/1  "PRBSNumPeriods"
  start/stop/1 -> Info Snapshot/Enable

== system ScanDc/Data Logging for 'frestimate'3/Generate Info Signal/Sinestream ==
  start/stop : Inport
  Info Bus : BusCreator  Inputs=1
  Info Snapshot : slctrl_fre/Frequency Response Estimator/Frequency Response Estimator/Variant Subsystem/PRBSNoEst/Info Snapshot  SystemSampleTime=-1  VariantActivationTime=update diagram  EmptyChoice=off  PassThrough=off  PassThroughVariantControl=(default)  EmptyChoiceVariantControl=(default)  AllowFlexibleInterface=on  Latency=0  AutoFrameSizeCalculation=off
  frequencies : Constant  Value=w  SampleTime=Ts
  Info : Outport
  wires:
  Info Snapshot/1 -> Info Bus/1  "frequencies"
  frequencies/1 -> Info Snapshot/1
  start/stop/1 -> Info Snapshot/Enable
  Info Bus/1 -> Info/1  "Info"

== system ScanDc/Data Logging for 'frestimate'3/Generate Ready Signal/PRBS ==
  Freq Index : Inport
  Perturbation : Inport  Port=2
  Constant : Constant  Value=0  SampleTime=Ts
  Relational Operator : RelationalOperator  Operator=~=  OutDataTypeStr=boolean  RndMeth=Simplest  InputSameDT=off
  Terminator : Terminator
  Ready : Outport
  wires:
  Relational Operator/1 -> Ready/1  "Ready"
  Constant/1 -> Relational Operator/2
  Perturbation/1 -> Relational Operator/1  "Perturbation"
  Freq Index/1 -> Terminator/1

== system ScanDc/Data Logging for 'frestimate'3/Generate Ready Signal/Sinestream ==
  Freq Index : Inport
  Perturbation : Inport  Port=2
  ExtractReadySignal : Subsystem  mask(Extract Ready Signal){Ts=Ts, Frequencies=w, NumOfSetPeriod=1, NumOfEstPeriod=2}
      mask prompts: Ts "Sample Time (Ts)"; Frequencies "Frequencies Vector"; NumOfSetPeriod "Number of Settling Periods"; NumOfEstPeriod "Number of Estimation Periods"
      mask help: Extract ready signal for the Sinestream Signal Generator block for offline frequency response estimation.
      mask init:
      | nw = length(Frequencies);
  Terminator : Terminator
  Ready : Outport
  wires:
  Freq Index/1 -> ExtractReadySignal/1(Frequency Index)
  Perturbation/1 -> Terminator/1
  ExtractReadySignal/1(Ready Signal) -> Ready/1  "Ready"

== system ScanDc/Data Logging for 'frestimate'3/Subtract Nominal Values/Enabled Subsystem ==
  u : Inport
  y : Inport  Port=2
  start/stop : Inport  Port=3
  Enable : EnablePort
  ExtractNominalValues : Subsystem  mask(Remove Nominal Signal){Ts=Ts}
      mask prompts: Ts "Samplt Time (sec)"
      mask help: Remove nominal baseline signal from logged data.
  Sum : Sum  Inputs=|+-
  Sum1 : Sum  Inputs=-+|
  PlantInput : Outport
  PlantOutput : Outport  Port=2
  wires:
  Sum1/1 -> PlantOutput/1
  y/1 -> ExtractNominalValues/2(y), Sum1/2
  ExtractNominalValues/2(yNominal) -> Sum1/1
  u/1 -> ExtractNominalValues/1(u), Sum/1
  ExtractNominalValues/1(uNominal) -> Sum/2
  Sum/1 -> PlantInput/1
  start/stop/1 -> ExtractNominalValues/3(start/stop)

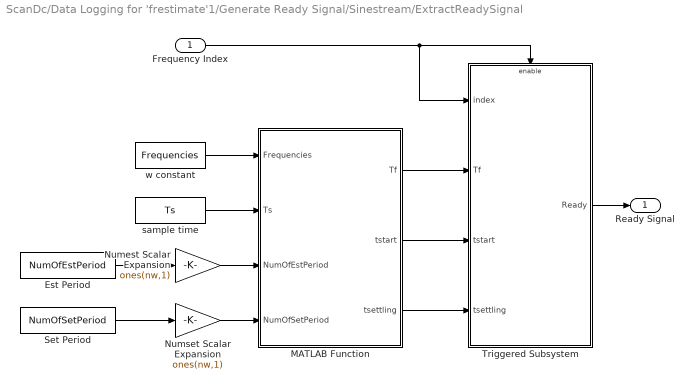
== system ScanDc/Data Logging for 'frestimate'1/Generate Ready Signal/Sinestream/ExtractReadySignal ==
  Frequency Index : Inport
  Est Period : Constant  Value=NumOfEstPeriod  OutDataTypeStr=double
  MATLAB Function : MATLAB Function  TreatAsAtomicUnit=on
  Numest Scalar Expansion : Gain  Gain=ones(nw,1)
  Numset Scalar Expansion : Gain  Gain=ones(nw,1)
  Set Period : Constant  Value=NumOfSetPeriod  OutDataTypeStr=double
  Triggered Subsystem : Subsystem  TreatAsAtomicUnit=on
  sample time : Constant  Value=Ts  OutDataTypeStr=double
  w constant : Constant  Value=Frequencies  OutDataTypeStr=double
  Ready Signal : Outport
  wires:
  MATLAB Function/3(tsettling) -> Triggered Subsystem/4(tsettling)
  MATLAB Function/2(tstart) -> Triggered Subsystem/3(tstart)
  Set Period/1 -> Numset Scalar Expansion/1
  Triggered Subsystem/1(Ready) -> Ready Signal/1
  Frequency Index/1 -> Triggered Subsystem/Enable, Triggered Subsystem/1(index)
  Numset Scalar Expansion/1 -> MATLAB Function/4(NumOfSetPeriod)
  Est Period/1 -> Numest Scalar Expansion/1
  MATLAB Function/1(Tf) -> Triggered Subsystem/2(Tf)
  w constant/1 -> MATLAB Function/1(Frequencies)
  Numest Scalar Expansion/1 -> MATLAB Function/3(NumOfEstPeriod)
  sample time/1 -> MATLAB Function/2(Ts)

== system ScanDc/Data Logging for 'frestimate'1/Subtract Nominal Values/Enabled Subsystem/ExtractNominalValues ==
  u : Inport
  y : Inport  Port=2
  start/stop : Inport  Port=3
  DisplayU0 : Display
  DisplayY0 : Display
  Enabled Delay U : Delay  DelayLength=1  InitialConditionSource=Input port  ExternalReset=Rising  SampleTime=Ts
      settings: InputPortMap=u0,r5,p4
  Enabled Delay Y : Delay  DelayLength=1  InitialConditionSource=Input port  ExternalReset=Rising  SampleTime=Ts
      settings: InputPortMap=u0,r5,p4
  uNominal : Outport  OutDataTypeStr=double  VectorParamsAs1DForOutWhenUnconnected=off
  yNominal : Outport  Port=2  OutDataTypeStr=double  VectorParamsAs1DForOutWhenUnconnected=off
  wires:
  y/1 -> Enabled Delay Y/3
  u/1 -> Enabled Delay U/3
  start/stop/1 -> Enabled Delay U/2, Enabled Delay Y/2
  Enabled Delay Y/1 -> DisplayY0/1, Enabled Delay Y/1, yNominal/1  "y"
  Enabled Delay U/1 -> Enabled Delay U/1, DisplayU0/1, uNominal/1  "u"

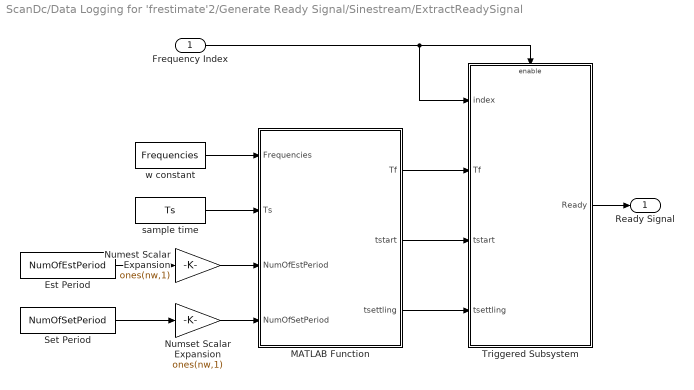
== system ScanDc/Data Logging for 'frestimate'2/Generate Ready Signal/Sinestream/ExtractReadySignal ==
  Frequency Index : Inport
  Est Period : Constant  Value=NumOfEstPeriod  OutDataTypeStr=double
  MATLAB Function : MATLAB Function  TreatAsAtomicUnit=on
  Numest Scalar Expansion : Gain  Gain=ones(nw,1)
  Numset Scalar Expansion : Gain  Gain=ones(nw,1)
  Set Period : Constant  Value=NumOfSetPeriod  OutDataTypeStr=double
  Triggered Subsystem : Subsystem  TreatAsAtomicUnit=on
  sample time : Constant  Value=Ts  OutDataTypeStr=double
  w constant : Constant  Value=Frequencies  OutDataTypeStr=double
  Ready Signal : Outport
  wires:
  MATLAB Function/3(tsettling) -> Triggered Subsystem/4(tsettling)
  MATLAB Function/2(tstart) -> Triggered Subsystem/3(tstart)
  Set Period/1 -> Numset Scalar Expansion/1
  Triggered Subsystem/1(Ready) -> Ready Signal/1
  Frequency Index/1 -> Triggered Subsystem/Enable, Triggered Subsystem/1(index)
  Numset Scalar Expansion/1 -> MATLAB Function/4(NumOfSetPeriod)
  Est Period/1 -> Numest Scalar Expansion/1
  MATLAB Function/1(Tf) -> Triggered Subsystem/2(Tf)
  w constant/1 -> MATLAB Function/1(Frequencies)
  Numest Scalar Expansion/1 -> MATLAB Function/3(NumOfEstPeriod)
  sample time/1 -> MATLAB Function/2(Ts)

== system ScanDc/Data Logging for 'frestimate'2/Subtract Nominal Values/Enabled Subsystem/ExtractNominalValues ==
  u : Inport
  y : Inport  Port=2
  start/stop : Inport  Port=3
  DisplayU0 : Display
  DisplayY0 : Display
  Enabled Delay U : Delay  DelayLength=1  InitialConditionSource=Input port  ExternalReset=Rising  SampleTime=Ts
      settings: InputPortMap=u0,r5,p4
  Enabled Delay Y : Delay  DelayLength=1  InitialConditionSource=Input port  ExternalReset=Rising  SampleTime=Ts
      settings: InputPortMap=u0,r5,p4
  uNominal : Outport  OutDataTypeStr=double  VectorParamsAs1DForOutWhenUnconnected=off
  yNominal : Outport  Port=2  OutDataTypeStr=double  VectorParamsAs1DForOutWhenUnconnected=off
  wires:
  y/1 -> Enabled Delay Y/3
  u/1 -> Enabled Delay U/3
  start/stop/1 -> Enabled Delay U/2, Enabled Delay Y/2
  Enabled Delay Y/1 -> DisplayY0/1, Enabled Delay Y/1, yNominal/1  "y"
  Enabled Delay U/1 -> Enabled Delay U/1, DisplayU0/1, uNominal/1  "u"

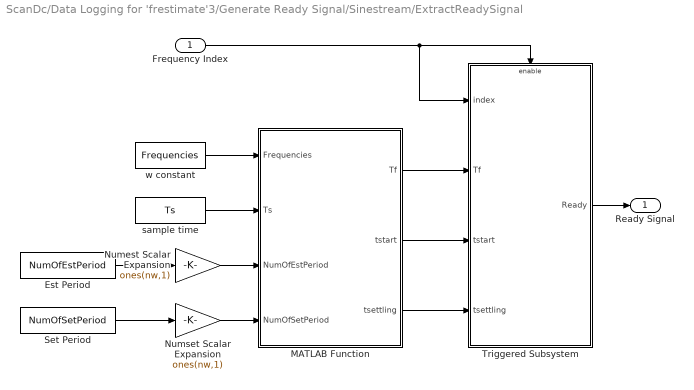
== system ScanDc/Data Logging for 'frestimate'3/Generate Ready Signal/Sinestream/ExtractReadySignal ==
  Frequency Index : Inport
  Est Period : Constant  Value=NumOfEstPeriod  OutDataTypeStr=double
  MATLAB Function : MATLAB Function  TreatAsAtomicUnit=on
  Numest Scalar Expansion : Gain  Gain=ones(nw,1)
  Numset Scalar Expansion : Gain  Gain=ones(nw,1)
  Set Period : Constant  Value=NumOfSetPeriod  OutDataTypeStr=double
  Triggered Subsystem : Subsystem  TreatAsAtomicUnit=on
  sample time : Constant  Value=Ts  OutDataTypeStr=double
  w constant : Constant  Value=Frequencies  OutDataTypeStr=double
  Ready Signal : Outport
  wires:
  MATLAB Function/3(tsettling) -> Triggered Subsystem/4(tsettling)
  MATLAB Function/2(tstart) -> Triggered Subsystem/3(tstart)
  Set Period/1 -> Numset Scalar Expansion/1
  Triggered Subsystem/1(Ready) -> Ready Signal/1
  Frequency Index/1 -> Triggered Subsystem/Enable, Triggered Subsystem/1(index)
  Numset Scalar Expansion/1 -> MATLAB Function/4(NumOfSetPeriod)
  Est Period/1 -> Numest Scalar Expansion/1
  MATLAB Function/1(Tf) -> Triggered Subsystem/2(Tf)
  w constant/1 -> MATLAB Function/1(Frequencies)
  Numest Scalar Expansion/1 -> MATLAB Function/3(NumOfEstPeriod)
  sample time/1 -> MATLAB Function/2(Ts)

== system ScanDc/Data Logging for 'frestimate'3/Subtract Nominal Values/Enabled Subsystem/ExtractNominalValues ==
  u : Inport
  y : Inport  Port=2
  start/stop : Inport  Port=3
  DisplayU0 : Display
  DisplayY0 : Display
  Enabled Delay U : Delay  DelayLength=1  InitialConditionSource=Input port  ExternalReset=Rising  SampleTime=Ts
      settings: InputPortMap=u0,r5,p4
  Enabled Delay Y : Delay  DelayLength=1  InitialConditionSource=Input port  ExternalReset=Rising  SampleTime=Ts
      settings: InputPortMap=u0,r5,p4
  uNominal : Outport  OutDataTypeStr=double  VectorParamsAs1DForOutWhenUnconnected=off
  yNominal : Outport  Port=2  OutDataTypeStr=double  VectorParamsAs1DForOutWhenUnconnected=off
  wires:
  y/1 -> Enabled Delay Y/3
  u/1 -> Enabled Delay U/3
  start/stop/1 -> Enabled Delay U/2, Enabled Delay Y/2
  Enabled Delay Y/1 -> DisplayY0/1, Enabled Delay Y/1, yNominal/1  "y"
  Enabled Delay U/1 -> Enabled Delay U/1, DisplayU0/1, uNominal/1  "u"

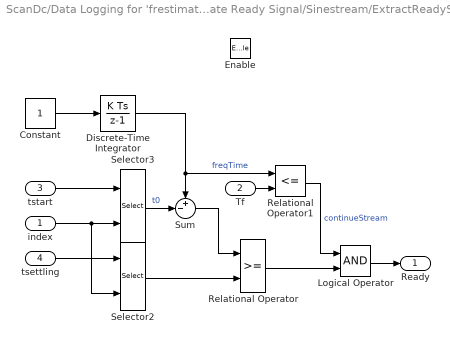
== system ScanDc/Data Logging for 'frestimate'1/Generate Ready Signal/Sinestream/ExtractReadySignal/Triggered Subsystem ==
  index : Inport
  Tf : Inport  Port=2
  tstart : Inport  Port=3
  tsettling : Inport  Port=4
  Enable : EnablePort
  Constant : Constant  OutDataTypeStr=double
  Discrete-Time Integrator : DiscreteIntegrator  SampleTime=Ts  ICPrevOutput=DiscIntNeverNeededParam  ICPrevScaledInput=DiscIntNeverNeededParam
  Logical Operator : Logic  AllPortsSameDT=off  OutDataTypeStr=boolean
  Relational Operator : RelationalOperator  OutDataTypeStr=boolean  RndMeth=Simplest  InputSameDT=off
  Relational Operator1 : RelationalOperator  Operator=<=  OutDataTypeStr=boolean  RndMeth=Simplest  InputSameDT=off
  Selector2 : Selector  InputPortWidth=nw  IndexOptions=Index vector (port)  Indices=[1 3]  OutputSizes=1
  Selector3 : Selector  InputPortWidth=nw  IndexOptions=Index vector (port)  Indices=[1 3]  OutputSizes=1
  Sum : Sum  Inputs=+-|
  Ready : Outport
  wires:
  Logical Operator/1 -> Ready/1
  Relational Operator1/1 -> Logical Operator/1  "continueStream"
  Tf/1 -> Relational Operator1/2
  Relational Operator/1 -> Logical Operator/2
  index/1 -> Selector3/2, Selector2/2
  Discrete-Time Integrator/1 -> Relational Operator1/1, Sum/1  "freqTime"
  Selector3/1 -> Sum/2  "t0"
  Selector2/1 -> Relational Operator/2
  tsettling/1 -> Selector2/1
  tstart/1 -> Selector3/1
  Sum/1 -> Relational Operator/1
  Constant/1 -> Discrete-Time Integrator/1
